simulink model "Kundur_BESS_STA_Nov14_2021a_v2_2021a"  (R2023a)
settings: Solver=VariableStepAuto  StartTime=0.0  StopTime=3  FixedStep=Ts  MaxStep=1e-5  MinStep=1e-20  RelTol=1e-3  EnableMultiTasking=on
PreLoadFcn:
  | Ts=50e-6;
PostLoadFcn:
  | Ts=50e-6;
InitFcn:
  | Ts=50e-6;
values from neighbouring files (symbols this model uses):
  current_K_den = [1 -1.95396088137 0.953960881373]    [param_cntrl_v2.mat]
  current_K_num = [292.549944556 -582.765243791 290.215658722]    [param_cntrl_v2.mat]
  flt_den = [1 -1.99914493247 0.999500180349]    [param_cntrl_v2.mat]
  flt_num = [0.000249925443627 3.12366678454e-08 -0.000249894206959]    [param_cntrl_v2.mat]
  flt_rocof_den = [1 -3.94812243331 5.84544117496 -3.84650440967 0.949185710471]    [param_cntrl_v2.mat]
  flt_rocof_num = [2.65341753303e-09 1.06136701321e-08 1.59205051982e-08 1.06136701321e-08 2.65341753303e-09]    [param_cntrl_v2.mat]
  pll_K_den = [1 -1.95396088137 0.953960881373]    [param_cntrl_v2.mat]
  pll_K_num = [1047.77474974 -2078.89023245 1031.12061217]    [param_cntrl_v2.mat]
  sampling_k = 5e-05    [param_cntrl_v2.mat]
undefined symbols (not defined in the file or in its folder): Ad2, Ad4, Bd2, Bd4, Cd2, Cd4, D1, Delta, flt_rocof_a_den, flt_rocof_a_num, flt_rocof_b_den, flt_rocof_b_num, Gd2, Gd4, Kd2, Kd4, L, R
libraries: spsThreePhaseVIMeasurementLib x15, spsLoadFlowBusLib x12, spsSeriesRLCBranchLib x11, spsThreePhaseSeriesRLCLoadLib x11, spsThreePhaseTransformerTwoWindingsLib x8, spsThreePhaseSeriesRLCBranchLib x8, spsabctoAlphaBetaZeroLib x8, spsGenericPowerSystemStabilizerLib x8, spsPowerPositiveSequenceLib x7, spsThreePhaseParallelRLCLoadLib x6, spsPLL3phLib x6, spsGroundLib x6
(part 4 of 4)

== system Kundur_BESS_STA_Nov14_2021a_v2_2021a/Area 2/sig1 ==
  In1 : Inport
  Bus Selector1 : BusSelector  OutputSignals="dq0 components.Stator voltage  vq (pu),dq0 components.Stator voltage  vd (pu),Mechanical.Rotor angle deviation  d_theta (rad),Mechanical.Rotor speed  wm  (pu),Mechanical.Electrical power  Pe (pu),Mechanical.Rotor speed deviation  dw (pu),Mechanical.Rotor mechanical angle  theta (deg)"
  Mux : Mux  Inputs=6
  Mux1 : Mux  Inputs=2
  Out1 : Outport  VectorParamsAs1DForOutWhenUnconnected=off
  wires:
  Mux1/1 -> Mux/1
  Bus Selector1/1 -> Mux1/1  "<Stator voltage  vq (pu)>"
  Bus Selector1/2 -> Mux1/2  "<Stator voltage  vd (pu)>"
  Bus Selector1/3 -> Mux/2  "<Rotor angle deviation  d_theta (rad)>"
  Bus Selector1/4 -> Mux/3  "<Rotor speed  wm  (pu)>"
  Bus Selector1/5 -> Mux/4  "<Electrical power  Pe (pu)>"
  Bus Selector1/6 -> Mux/5  "<Rotor speed deviation  dw (pu)>"
  Bus Selector1/7 -> Mux/6  "<Rotor mechanical angle  theta (deg)>"
  In1/1 -> Bus Selector1/1
  Mux/1 -> Out1/1

== system Kundur_BESS_STA_Nov14_2021a_v2_2021a/Area 2/sig2 ==
  In1 : Inport
  Bus Selector1 : BusSelector  OutputSignals="dq0 components.Stator voltage  vq (pu),dq0 components.Stator voltage  vd (pu),Mechanical.Rotor angle deviation  d_theta (rad),Mechanical.Rotor speed  wm  (pu),Mechanical.Electrical power  Pe (pu),Mechanical.Rotor speed deviation  dw (pu),Mechanical.Rotor mechanical angle  theta (deg)"
  Mux : Mux  Inputs=6
  Mux1 : Mux  Inputs=2
  Out1 : Outport  VectorParamsAs1DForOutWhenUnconnected=off
  wires:
  Mux1/1 -> Mux/1
  Bus Selector1/1 -> Mux1/1  "<Stator voltage  vq (pu)>"
  Bus Selector1/2 -> Mux1/2  "<Stator voltage  vd (pu)>"
  Bus Selector1/3 -> Mux/2  "<Rotor angle deviation  d_theta (rad)>"
  Bus Selector1/4 -> Mux/3  "<Rotor speed  wm  (pu)>"
  Bus Selector1/5 -> Mux/4  "<Electrical power  Pe (pu)>"
  Bus Selector1/6 -> Mux/5  "<Rotor speed deviation  dw (pu)>"
  Bus Selector1/7 -> Mux/6  "<Rotor mechanical angle  theta (deg)>"
  In1/1 -> Bus Selector1/1
  Mux/1 -> Out1/1

== system Kundur_BESS_STA_Nov14_2021a_v2_2021a/Area 1/BESS/Subsystem ==
  note: Alpha-Beta-Zero
      | to abc
  dq0 : Inport  PortDimensions=3
  wt1 : Inport  Port=2  PortDimensions=1
  Alpha-Beta-Zero to abc : spsAlphaBetaZerotoabcLib/Alpha-Beta-Zero to abc
  DQ to Alpha beta : Subsystem
  abc : Outport  VectorParamsAs1DForOutWhenUnconnected=off
  wires:
  Alpha-Beta-Zero to abc/1 -> abc/1
  dq0/1 -> DQ to Alpha beta/1(dq0)
  DQ to Alpha beta/1(al_be_0) -> Alpha-Beta-Zero to abc/1
  wt1/1 -> DQ to Alpha beta/2(wt1)

== system Kundur_BESS_STA_Nov14_2021a_v2_2021a/Area 1/BESS/Subsystem1 ==
  wt : Inport  PortDimensions=1
  abc : Inport  Port=2  PortDimensions=3
  Demux : Demux  Outputs=3
  Mux : Mux  Inputs=2
  Subsystem1 : Subsystem
  Terminator : Terminator
  abc to Alpha-Beta-Zero : spsabctoAlphaBetaZeroLib/abc to Alpha-Beta-Zero
  dq : Outport  VectorParamsAs1DForOutWhenUnconnected=off
  wires:
  Subsystem1/1(dq) -> dq/1
  abc/1 -> abc to Alpha-Beta-Zero/1
  wt/1 -> Subsystem1/2(wt1)
  Demux/1 -> Mux/1
  Demux/2 -> Mux/2
  Mux/1 -> Subsystem1/1(al_be)
  abc to Alpha-Beta-Zero/1 -> Demux/1
  Demux/3 -> Terminator/1

== system Kundur_BESS_STA_Nov14_2021a_v2_2021a/Area 1/BESS/Subsystem2 ==
  wt : Inport  PortDimensions=1
  abc : Inport  Port=2  PortDimensions=3
  Demux : Demux  Outputs=3
  Mux : Mux  Inputs=2
  Subsystem1 : Subsystem
  Terminator : Terminator
  abc to Alpha-Beta-Zero : spsabctoAlphaBetaZeroLib/abc to Alpha-Beta-Zero
  dq : Outport  VectorParamsAs1DForOutWhenUnconnected=off
  wires:
  Subsystem1/1(dq) -> dq/1
  abc/1 -> abc to Alpha-Beta-Zero/1
  wt/1 -> Subsystem1/2(wt1)
  Demux/1 -> Mux/1
  Demux/2 -> Mux/2
  Demux/3 -> Terminator/1
  Mux/1 -> Subsystem1/1(al_be)
  abc to Alpha-Beta-Zero/1 -> Demux/1

== system Kundur_BESS_STA_Nov14_2021a_v2_2021a/Area 1/BESS/Subsystem3 ==
  e(S) : Inport
  Add : Sum
  Integrator : Integrator
  Ki : Gain  Gain=Ki
  Kp : Gain  Gain=Kp
  u(S) : Outport  VectorParamsAs1DForOutWhenUnconnected=off
  wires:
  Kp/1 -> Add/1
  e(S)/1 -> Ki/1, Kp/1
  Ki/1 -> Integrator/1
  Add/1 -> u(S)/1  "u(S)"
  Integrator/1 -> Add/2

== system Kundur_BESS_STA_Nov14_2021a_v2_2021a/Area 1/BESS/Subsystem4 ==
  e(S) : Inport
  Add : Sum
  Integrator : Integrator
  Ki : Gain  Gain=Ki
  Kp : Gain  Gain=Kp
  u(S) : Outport  VectorParamsAs1DForOutWhenUnconnected=off
  wires:
  Kp/1 -> Add/1
  e(S)/1 -> Ki/1, Kp/1
  Ki/1 -> Integrator/1
  Add/1 -> u(S)/1  "u(S)"
  Integrator/1 -> Add/2

== system Kundur_BESS_STA_Nov14_2021a_v2_2021a/Area 1/BESS2 /Subsystem ==
  note: Alpha-Beta-Zero
      | to abc
  dq0 : Inport  PortDimensions=3
  wt1 : Inport  Port=2  PortDimensions=1
  Alpha-Beta-Zero to abc : spsAlphaBetaZerotoabcLib/Alpha-Beta-Zero to abc
  DQ to Alpha beta : Subsystem
  abc : Outport  VectorParamsAs1DForOutWhenUnconnected=off
  wires:
  Alpha-Beta-Zero to abc/1 -> abc/1
  dq0/1 -> DQ to Alpha beta/1(dq0)
  DQ to Alpha beta/1(al_be_0) -> Alpha-Beta-Zero to abc/1
  wt1/1 -> DQ to Alpha beta/2(wt1)

== system Kundur_BESS_STA_Nov14_2021a_v2_2021a/Area 1/BESS2 /Subsystem1 ==
  wt : Inport  PortDimensions=1
  abc : Inport  Port=2  PortDimensions=3
  Demux : Demux  Outputs=3
  Mux : Mux  Inputs=2
  Subsystem1 : Subsystem
  Terminator : Terminator
  abc to Alpha-Beta-Zero : spsabctoAlphaBetaZeroLib/abc to Alpha-Beta-Zero
  dq : Outport  VectorParamsAs1DForOutWhenUnconnected=off
  wires:
  Subsystem1/1(dq) -> dq/1
  abc/1 -> abc to Alpha-Beta-Zero/1
  wt/1 -> Subsystem1/2(wt1)
  Demux/1 -> Mux/1
  Demux/2 -> Mux/2
  Mux/1 -> Subsystem1/1(al_be)
  abc to Alpha-Beta-Zero/1 -> Demux/1
  Demux/3 -> Terminator/1

== system Kundur_BESS_STA_Nov14_2021a_v2_2021a/Area 1/BESS2 /Subsystem2 ==
  wt : Inport  PortDimensions=1
  abc : Inport  Port=2  PortDimensions=3
  Demux : Demux  Outputs=3
  Mux : Mux  Inputs=2
  Subsystem1 : Subsystem
  Terminator : Terminator
  abc to Alpha-Beta-Zero : spsabctoAlphaBetaZeroLib/abc to Alpha-Beta-Zero
  dq : Outport  VectorParamsAs1DForOutWhenUnconnected=off
  wires:
  Subsystem1/1(dq) -> dq/1
  abc/1 -> abc to Alpha-Beta-Zero/1
  wt/1 -> Subsystem1/2(wt1)
  Demux/1 -> Mux/1
  Demux/2 -> Mux/2
  Demux/3 -> Terminator/1
  Mux/1 -> Subsystem1/1(al_be)
  abc to Alpha-Beta-Zero/1 -> Demux/1

== system Kundur_BESS_STA_Nov14_2021a_v2_2021a/Area 1/BESS2 /Subsystem3 ==
  e(S) : Inport
  Add : Sum
  Integrator : Integrator
  Ki : Gain  Gain=Ki
  Kp : Gain  Gain=Kp
  u(S) : Outport  VectorParamsAs1DForOutWhenUnconnected=off
  wires:
  Kp/1 -> Add/1
  e(S)/1 -> Ki/1, Kp/1
  Ki/1 -> Integrator/1
  Add/1 -> u(S)/1  "u(S)"
  Integrator/1 -> Add/2

== system Kundur_BESS_STA_Nov14_2021a_v2_2021a/Area 1/BESS2 /Subsystem4 ==
  e(S) : Inport
  Add : Sum
  Integrator : Integrator
  Ki : Gain  Gain=Ki
  Kp : Gain  Gain=Kp
  u(S) : Outport  VectorParamsAs1DForOutWhenUnconnected=off
  wires:
  Kp/1 -> Add/1
  e(S)/1 -> Ki/1, Kp/1
  Ki/1 -> Integrator/1
  Add/1 -> u(S)/1  "u(S)"
  Integrator/1 -> Add/2

== system Kundur_BESS_STA_Nov14_2021a_v2_2021a/Area 2/BESS/Aver. Inverter ==
  U_abc : Inport
  Controlled Voltage Source : spsControlledVoltageSourceLib/Controlled Voltage Source  Initialize=on  Source_Type=AC  Amplitude=0  Phase=0  Frequency=0  Measurements=None
  Controlled Voltage Source1 : spsControlledVoltageSourceLib/Controlled Voltage Source  Initialize=on  Source_Type=AC  Amplitude=0  Phase=0  Frequency=0  Measurements=None
  Controlled Voltage Source2 : spsControlledVoltageSourceLib/Controlled Voltage Source  Initialize=on  Source_Type=AC  Amplitude=0  Phase=0  Frequency=0  Measurements=None
  Demux : Demux  Outputs=3
  Ground : spsGroundLib/Ground  LConnTagsString=a
  A : PMIOPort  Side=Right
  B : PMIOPort  Port=2  Side=Right
  C : PMIOPort  Port=3  Side=Right
  wires:
  Demux/1 -> Controlled Voltage Source/1
  Demux/2 -> Controlled Voltage Source1/1
  Demux/3 -> Controlled Voltage Source2/1
  U_abc/1 -> Demux/1
  connections:
  Controlled Voltage Source/LConn1 -- Controlled Voltage Source1/LConn1 -- Controlled Voltage Source2/LConn1 -- Ground/LConn1
  Controlled Voltage Source2/RConn1 -- C/RConn1
  Controlled Voltage Source1/RConn1 -- B/RConn1
  Controlled Voltage Source/RConn1 -- A/RConn1

== system Kundur_BESS_STA_Nov14_2021a_v2_2021a/Area 2/BESS/I_ref ==
  note: Ud^2+Uq^2
  note: [Uq;Ud]
  note: [Ud;-Uq]
  PQ : Inport
  U_dq0 : Inport  Port=2
  Constant : Constant  Value=0
  Divide : Product  Inputs=*/
  Divide1 : Product  Inputs=*/
  Dot Product : DotProduct  OutDataTypeStr=Inherit: Inherit via internal rule
  Dot Product1 : DotProduct  OutDataTypeStr=Inherit: Inherit via internal rule
  Dot Product2 : DotProduct  OutDataTypeStr=Inherit: Inherit via internal rule
  Gain : Gain  Gain=[1,0;0,-1]  Multiplication=Matrix(K*u)
  Gain1 : Gain  Gain=[0,1;1,0]  Multiplication=Matrix(K*u)
  Gain2 : Gain  Gain=2/3
  Gain3 : Gain  Gain=2/3
  Mux : Mux  Inputs=3
  Saturation : Saturate  UpperLimit=1e10  LowerLimit=1e-4
  Selector : Selector  InputPortWidth=3  IndexOptions=Index vector (dialog)  Indices=[1 2]  OutputSizes=1
  I_dq0_ref : Outport
  wires:
  U_dq0/1 -> Selector/1
  Selector/1 -> Dot Product2/1, Dot Product2/2, Gain1/1, Gain/1
  Gain/1 -> Dot Product/2
  Gain1/1 -> Dot Product1/2
  PQ/1 -> Dot Product/1, Dot Product1/1
  Dot Product/1 -> Divide/1
  Dot Product1/1 -> Divide1/1
  Divide/1 -> Gain2/1
  Divide1/1 -> Gain3/1
  Mux/1 -> I_dq0_ref/1
  Constant/1 -> Mux/3
  Dot Product2/1 -> Saturation/1
  Saturation/1 -> Divide1/2, Divide/2
  Gain2/1 -> Mux/1
  Gain3/1 -> Mux/2

== system Kundur_BESS_STA_Nov14_2021a_v2_2021a/Area 2/BESS/SRF-PLL1 ==
  Uabc : Inport
  Alpha-Beta-Zero to dq0 : spsAlphaBetaZerotodq0Lib/Alpha-Beta-Zero to dq0  Alignment=Aligned with phase A axis
  Constant1 : Constant  Value=60*2*pi
  DSOGI : Subsystem  Commented=on
      settings: PortSchema="{\"entries\":[{\"content\":{\"sides\":[{\"content\":{\"connectorIds\":[\"In1\"]},\"type\":\"ConnectorPlacement.EquallySpacedRectSide\",\"uuid\":\"0e58ca25-f6ec-443d-b264-f69bb116b758\"},{\"content\":{\"connectorIds\":[\"Out1\"],\"side\":\"RIGHT\"},\"type\":\"ConnectorPlacement.EquallySpacedRectSide\",\"uuid\":\"f4052289-4772-41c6-aa5a-e32d1aa36c69\"},{\"content\":{\"side\":\"TOP\"},\"type\":\"ConnectorPlacement.EquallySpacedRectSide\",\"uuid\":\"ea46d89b-d5cb-4111-9a8a-24f542a45993\"},{\"content\":{\"connectorIds\":[\"In2\"],\"side\":\"BOTTOM\"},\"type\":\"ConnectorPlacement.EquallySpacedRectSide\",\"uuid\":\"bc0e78b7-d9b3-48dd-a6ae-aa9871795585\"}]},\"type\":\"ConnectorPlacement.EquallySpacedConnector\",\"uuid\":\"463a5158-fade-4a5a-b60d-59d7cf065d44\"}],\"packageUris\":[\"http://schema.mathworks.com/mf0/Connector/R2020b\"],\"version\":\"1.0\"}"
  Discrete Transfer Fcn : DiscreteTransferFcn  Numerator=pll_K_num  Denominator=pll_K_den
  Filter : Subsystem  Commented=on
  Gain : Gain  Gain=sampling_k
  Normalization : dspmathops/Normalization  NormType=2-norm  Bias=1e-10  NormOver=Each column  Dimension=1  roundingMode=Floor  overflowMode=off  accumDataTypeStr=Inherit: Same as product output  accumLastDataTypeStr=Inherit: Same as product output  outputDataTypeStr=Inherit: Same as product output  outputMin=[]  outputMax=[]  outputLastDataTypeStr=Inherit: Same as product output
  Quadrature : Subsystem
  Scope : Scope
  Selector : Selector  InputPortWidth=3  IndexOptions=Index vector (dialog)  Indices=2  OutputSizes=1
  Sum : Sum  Inputs=++|
  Sum2 : Sum  Inputs=++|
  Unit Delay : UnitDelay  SampleTime=sampling_k  HasFrameUpgradeWarning=on
  Wrap : Subsystem
  filt : Subsystem
  w : Outport
  ph : Outport  Port=2
  wires:
  Sum/1 -> Unit Delay/1
  Gain/1 -> Sum/2
  Unit Delay/1 -> Wrap/1(phi)
  Selector/1 -> Scope/1, Discrete Transfer Fcn/1
  Discrete Transfer Fcn/1 -> Sum2/2
  Sum2/1 -> filt/1(u), Gain/1
  Constant1/1 -> Sum2/1
  Alpha-Beta-Zero to dq0/1 -> Selector/1
  Normalization/1 -> Alpha-Beta-Zero to dq0/1
  Quadrature/1(Ualphbet0) -> Normalization/1
  Uabc/1 -> Quadrature/1(Uabc)
  filt/1(uf) -> Quadrature/2(w), w/1
  Wrap/1(w_phi) -> ph/1, Alpha-Beta-Zero to dq0/2, Sum/1

== system Kundur_BESS_STA_Nov14_2021a_v2_2021a/Area 2/BESS/Support Control ==
  note: 1) Add Subsystem or Model blocks as valid variant choices.
      | 2) You cannot connect blocks at this level. At simulation, connectivity is automatically
      | determined, based on the active variant and port name matching.
  Vabc : Inport
  Gains : Inport  Port=2
  Droop (Proportional) : Subsystem  VariantControl=false
  VI with Diff : Subsystem  VariantControl=false
  VI with STA : Subsystem  VariantControl=true
  P_ref : Outport

== system Kundur_BESS_STA_Nov14_2021a_v2_2021a/Area 2/BESS/abc-to-dq0 ==
  Uabc : Inport
  Iabc : Inport  Port=2
  wt : Inport  Port=3
  abc to dq2 : spsabctodq0Lib/abc to dq0  Alignment=90 degrees behind phase A axis
  abc to dq3 : spsabctodq0Lib/abc to dq0  Alignment=90 degrees behind phase A axis
  Udq0 : Outport
  Idq0 : Outport  Port=2
  wires:
  wt/1 -> abc to dq3/2, abc to dq2/2
  Iabc/1 -> abc to dq3/1
  Uabc/1 -> abc to dq2/1
  abc to dq2/1 -> Udq0/1
  abc to dq3/1 -> Idq0/1

== system Kundur_BESS_STA_Nov14_2021a_v2_2021a/Area 1/BESS/Subsystem/DQ to Alpha beta ==
  dq0 : Inport  PortDimensions=3
  wt1 : Inport  Port=2  PortDimensions=1
  Demux4 : Demux  Outputs=[2 1]
  Fcn : Fcn  Expr=u[1]*sin(u[3]) + u[2]*cos(u[3])
  Fcn1 : Fcn  Expr=-u[1]*cos(u[3]) + u[2]*sin(u[3])
  Mux1 : Mux  Inputs=[2 1]
  Mux4 : Mux  Inputs=2
  Mux5 : Mux  Inputs=[2 1]
  Mux6 : Mux  Inputs=[2 1]
  al_be_0 : Outport  VectorParamsAs1DForOutWhenUnconnected=off
  wires:
  Mux4/1 -> Mux1/1
  Mux6/1 -> Fcn1/1
  Fcn1/1 -> Mux4/2
  Demux4/1 -> Mux6/1, Mux5/1
  Mux5/1 -> Fcn/1
  Demux4/2 -> Mux1/2
  Fcn/1 -> Mux4/1
  wt1/1 -> Mux5/2, Mux6/2
  dq0/1 -> Demux4/1
  Mux1/1 -> al_be_0/1

== system Kundur_BESS_STA_Nov14_2021a_v2_2021a/Area 1/BESS/Subsystem1/Subsystem1 ==
  note: q = al*cos(wt) + be*sin(wt)
  note: d = al*sin(wt) - be*cos(wt)
  al_be : Inport  PortDimensions=2
  wt1 : Inport  Port=2  PortDimensions=1
  Fcn : Fcn  Expr=u[1]*sin(u[3]) - u[2]*cos(u[3])
  Fcn1 : Fcn  Expr=u[1]*cos(u[3]) + u[2]*sin(u[3])
  Mux4 : Mux  Inputs=2
  Mux5 : Mux  Inputs=[2 1]
  Mux6 : Mux  Inputs=[2 1]
  dq : Outport  VectorParamsAs1DForOutWhenUnconnected=off
  wires:
  Mux5/1 -> Fcn/1
  Fcn1/1 -> Mux4/2
  al_be/1 -> Mux6/1, Mux5/1
  wt1/1 -> Mux5/2, Mux6/2
  Mux6/1 -> Fcn1/1
  Fcn/1 -> Mux4/1
  Mux4/1 -> dq/1

== system Kundur_BESS_STA_Nov14_2021a_v2_2021a/Area 1/BESS/Subsystem2/Subsystem1 ==
  note: q = al*cos(wt) + be*sin(wt)
  note: d = al*sin(wt) - be*cos(wt)
  al_be : Inport  PortDimensions=2
  wt1 : Inport  Port=2  PortDimensions=1
  Fcn : Fcn  Expr=u[1]*sin(u[3]) - u[2]*cos(u[3])
  Fcn1 : Fcn  Expr=u[1]*cos(u[3]) + u[2]*sin(u[3])
  Mux4 : Mux  Inputs=2
  Mux5 : Mux  Inputs=[2 1]
  Mux6 : Mux  Inputs=[2 1]
  dq : Outport  VectorParamsAs1DForOutWhenUnconnected=off
  wires:
  Mux5/1 -> Fcn/1
  Fcn1/1 -> Mux4/2
  al_be/1 -> Mux6/1, Mux5/1
  wt1/1 -> Mux5/2, Mux6/2
  Mux6/1 -> Fcn1/1
  Fcn/1 -> Mux4/1
  Mux4/1 -> dq/1

== system Kundur_BESS_STA_Nov14_2021a_v2_2021a/Area 1/BESS2 /Subsystem/DQ to Alpha beta ==
  dq0 : Inport  PortDimensions=3
  wt1 : Inport  Port=2  PortDimensions=1
  Demux4 : Demux  Outputs=[2 1]
  Fcn : Fcn  Expr=u[1]*sin(u[3]) + u[2]*cos(u[3])
  Fcn1 : Fcn  Expr=-u[1]*cos(u[3]) + u[2]*sin(u[3])
  Mux1 : Mux  Inputs=[2 1]
  Mux4 : Mux  Inputs=2
  Mux5 : Mux  Inputs=[2 1]
  Mux6 : Mux  Inputs=[2 1]
  al_be_0 : Outport  VectorParamsAs1DForOutWhenUnconnected=off
  wires:
  Mux4/1 -> Mux1/1
  Mux6/1 -> Fcn1/1
  Fcn1/1 -> Mux4/2
  Demux4/1 -> Mux6/1, Mux5/1
  Mux5/1 -> Fcn/1
  Demux4/2 -> Mux1/2
  Fcn/1 -> Mux4/1
  wt1/1 -> Mux5/2, Mux6/2
  dq0/1 -> Demux4/1
  Mux1/1 -> al_be_0/1

== system Kundur_BESS_STA_Nov14_2021a_v2_2021a/Area 1/BESS2 /Subsystem1/Subsystem1 ==
  note: q = al*cos(wt) + be*sin(wt)
  note: d = al*sin(wt) - be*cos(wt)
  al_be : Inport  PortDimensions=2
  wt1 : Inport  Port=2  PortDimensions=1
  Fcn : Fcn  Expr=u[1]*sin(u[3]) - u[2]*cos(u[3])
  Fcn1 : Fcn  Expr=u[1]*cos(u[3]) + u[2]*sin(u[3])
  Mux4 : Mux  Inputs=2
  Mux5 : Mux  Inputs=[2 1]
  Mux6 : Mux  Inputs=[2 1]
  dq : Outport  VectorParamsAs1DForOutWhenUnconnected=off
  wires:
  Mux5/1 -> Fcn/1
  Fcn1/1 -> Mux4/2
  al_be/1 -> Mux6/1, Mux5/1
  wt1/1 -> Mux5/2, Mux6/2
  Mux6/1 -> Fcn1/1
  Fcn/1 -> Mux4/1
  Mux4/1 -> dq/1

== system Kundur_BESS_STA_Nov14_2021a_v2_2021a/Area 1/BESS2 /Subsystem2/Subsystem1 ==
  note: q = al*cos(wt) + be*sin(wt)
  note: d = al*sin(wt) - be*cos(wt)
  al_be : Inport  PortDimensions=2
  wt1 : Inport  Port=2  PortDimensions=1
  Fcn : Fcn  Expr=u[1]*sin(u[3]) - u[2]*cos(u[3])
  Fcn1 : Fcn  Expr=u[1]*cos(u[3]) + u[2]*sin(u[3])
  Mux4 : Mux  Inputs=2
  Mux5 : Mux  Inputs=[2 1]
  Mux6 : Mux  Inputs=[2 1]
  dq : Outport  VectorParamsAs1DForOutWhenUnconnected=off
  wires:
  Mux5/1 -> Fcn/1
  Fcn1/1 -> Mux4/2
  al_be/1 -> Mux6/1, Mux5/1
  wt1/1 -> Mux5/2, Mux6/2
  Mux6/1 -> Fcn1/1
  Fcn/1 -> Mux4/1
  Mux4/1 -> dq/1

== system Kundur_BESS_STA_Nov14_2021a_v2_2021a/Area 2/BESS/SRF-PLL1/DSOGI ==
  Uabc : Inport
  w(t) : Inport  Port=2
  Constant : Constant  Value=0
  Gain : Gain  Gain=1/1000
  Gain1 : Gain  Gain=0.01
  Gain2 : Gain  Gain=0.01
  Integrator{,1..3} (4 alike) : Integrator
  Mux : Mux  Inputs=3
  Product{,1..3} (4 alike) : Product
  Selector1 : Selector  InputPortWidth=3  IndexOptions=Index vector (dialog)  Indices=1  OutputSizes=1
  Selector2 : Selector  InputPortWidth=3  IndexOptions=Index vector (dialog)  Indices=2  OutputSizes=1
  Sum1 : Sum  Inputs=-+|
  Sum2 : Sum  Inputs=|+-
  Sum3 : Sum  Inputs=-+|
  Sum4 : Sum  Inputs=|+-
  Sum5 : Sum  Inputs=|+-
  Sum6 : Sum  Inputs=|++
  Zero-Order Hold2 : ZeroOrderHold  SampleTime=sampling_k
  abc to Alpha-Beta-Zero : spsabctoAlphaBetaZeroLib/abc to Alpha-Beta-Zero
  Ualphbet0 : Outport
  wires:
  Sum4/1 -> Product/2
  Selector1/1 -> Sum1/2
  Gain/1 -> Selector2/1, Selector1/1
  Gain1/1 -> Sum4/1
  Sum1/1 -> Gain1/1
  Uabc/1 -> abc to Alpha-Beta-Zero/1
  Product/1 -> Integrator/1
  Product1/1 -> Integrator1/1
  Integrator1/1 -> [qv_alpha], Sum4/2
  Integrator/1 -> Product1/2, [v_alpha], Sum1/1, Sum2/1
  w(t)/1 -> Product2/1, Product3/1, Product1/1, Product/1
  Selector2/1 -> Sum3/2
  Sum3/1 -> Gain2/1
  Gain2/1 -> Sum5/1
  Sum5/1 -> Product2/2
  Product2/1 -> Integrator2/1
  Integrator2/1 -> [v_beta], Product3/2, Sum3/1, Sum6/1
  Product3/1 -> Integrator3/1
  Integrator3/1 -> [qv_beta], Sum5/2
  Sum2/1 -> Mux/1
  Sum6/1 -> Mux/2
  Constant/1 -> Mux/3
  Mux/1 -> Zero-Order Hold2/1
  Zero-Order Hold2/1 -> Ualphbet0/1
  abc to Alpha-Beta-Zero/1 -> Gain/1
  [qv_beta] -> Sum2/2
  [qv_alpha] -> Sum6/2

== system Kundur_BESS_STA_Nov14_2021a_v2_2021a/Area 2/BESS/SRF-PLL1/Filter ==
  Uabc : Inport
  Demux : Demux  Outputs=3
  Discrete Transfer Fcn : DiscreteTransferFcn  Numerator=flt_num  Denominator=flt_den
  Discrete Transfer Fcn1 : DiscreteTransferFcn  Numerator=flt_num  Denominator=flt_den
  Discrete Transfer Fcn2 : DiscreteTransferFcn  Numerator=flt_num  Denominator=flt_den
  Mux : Mux  Inputs=3
  Zero-Order Hold1 : ZeroOrderHold  SampleTime=sampling_k
  Zero-Order Hold2 : ZeroOrderHold  SampleTime=sampling_k
  Zero-Order Hold3 : ZeroOrderHold  SampleTime=sampling_k
  Uabc_f : Outport
  wires:
  Uabc/1 -> Demux/1
  Mux/1 -> Uabc_f/1
  Demux/1 -> Zero-Order Hold2/1
  Demux/2 -> Zero-Order Hold1/1
  Demux/3 -> Zero-Order Hold3/1
  Zero-Order Hold2/1 -> Discrete Transfer Fcn/1
  Zero-Order Hold1/1 -> Discrete Transfer Fcn1/1
  Zero-Order Hold3/1 -> Discrete Transfer Fcn2/1
  Discrete Transfer Fcn/1 -> Mux/1
  Discrete Transfer Fcn1/1 -> Mux/2
  Discrete Transfer Fcn2/1 -> Mux/3

== system Kundur_BESS_STA_Nov14_2021a_v2_2021a/Area 2/BESS/SRF-PLL1/Quadrature ==
  Uabc : Inport
  w : Inport  Port=2
  Constant : Constant  Value=0
  Divide : Product  Inputs=*/
  Gain : Gain  Gain=1/1000
  Mux : Mux  Inputs=3
  Saturation : Saturate  UpperLimit=62*2*pi  LowerLimit=59*2*pi
  Scope1 : Scope  NumInputPorts=2
  Selector : Selector  InputPortWidth=3  IndexOptions=Index vector (dialog)  Indices=1  OutputSizes=1
  State-Space : StateSpace  A=[-42e3,1,0;-586e6,0,1;-2712e9,0,0]  B=[42e3;586e6;2712e9]  C=[0,1,0]  D=[0]  InitialCondition=0
  Transfer Fcn1 : TransferFcn  Denominator=[1/(1200*2*pi)^2,2*0.1/(1200*2*pi),1]
  Zero-Order Hold2 : ZeroOrderHold  SampleTime=sampling_k
  abc to Alpha-Beta-Zero : spsabctoAlphaBetaZeroLib/abc to Alpha-Beta-Zero
  Ualphbet0 : Outport
  wires:
  Uabc/1 -> Gain/1
  Gain/1 -> abc to Alpha-Beta-Zero/1
  Zero-Order Hold2/1 -> Ualphbet0/1
  abc to Alpha-Beta-Zero/1 -> Selector/1
  Constant/1 -> Mux/3
  Mux/1 -> Zero-Order Hold2/1
  Transfer Fcn1/1 -> Scope1/2, Mux/2, State-Space/1
  State-Space/1 -> Divide/1
  w/1 -> Saturation/1
  Saturation/1 -> Divide/2
  Divide/1 -> Scope1/1, Mux/1
  Selector/1 -> Transfer Fcn1/1

== system Kundur_BESS_STA_Nov14_2021a_v2_2021a/Area 2/BESS/SRF-PLL1/Wrap ==
  phi : Inport
  Constant : Constant  Value=pi
  Constant1 : Constant  Value=2*pi
  Divide : Product  Inputs=*/
  Floor : Rounding
  Product : Product
  Sum : Sum  Inputs=|+-
  Sum1 : Sum  Inputs=|+-
  Sum2 : Sum  Inputs=|+-
  w_phi : Outport
  wires:
  phi/1 -> Sum/1
  Constant/1 -> Sum2/2, Sum/2
  Sum/1 -> Divide/1, Sum1/1
  Constant1/1 -> Product/2, Divide/2
  Divide/1 -> Floor/1
  Floor/1 -> Product/1
  Product/1 -> Sum1/2
  Sum1/1 -> Sum2/1
  Sum2/1 -> w_phi/1

== system Kundur_BESS_STA_Nov14_2021a_v2_2021a/Area 2/BESS/SRF-PLL1/filt ==
  u : Inport
  Discrete Transfer Fcn1 : DiscreteTransferFcn  Numerator=flt_rocof_num  Denominator=flt_rocof_den
  Discrete Transfer Fcn2 : DiscreteTransferFcn  Numerator=flt_rocof_num  Denominator=flt_rocof_den
  uf : Outport
  wires:
  u/1 -> Discrete Transfer Fcn1/1
  Discrete Transfer Fcn1/1 -> Discrete Transfer Fcn2/1
  Discrete Transfer Fcn2/1 -> uf/1

== system Kundur_BESS_STA_Nov14_2021a_v2_2021a/Area 2/BESS/Support Control/Droop (Proportional) ==
  Vabc : Inport
  Gains : Inport  Port=2
  Gain : Gain  Gain=-1
  PLL (3ph) : spsPLL3phLib/PLL (3ph)  Fmin=45  Par_Init=[0, 50]  ParK=[180, 3200, 0]  TcD=1e-4  MaxRateChangeFreq=12  FilterCutOffFreq=25  Ts=0  AGC=on
  Product : Product
  Selector : Selector  InputPortWidth=3  IndexOptions=Index vector (dialog)  Indices=1  OutputSizes=1
  Selector1 : Selector  InputPortWidth=3  IndexOptions=Index vector (dialog)  Indices=3  OutputSizes=1
  Sum : Sum  Inputs=-+|
  Terminator : Terminator
  P_ref : Outport
  wires:
  Vabc/1 -> PLL (3ph)/1
  Gains/1 -> Selector1/1, Selector/1
  PLL (3ph)/1 -> Sum/2  "freq"
  Selector1/1 -> Sum/1  "freq 0"
  PLL (3ph)/2 -> Terminator/1
  Sum/1 -> Product/2
  Selector/1 -> Product/1  "K_P"
  Product/1 -> Gain/1
  Gain/1 -> P_ref/1

== system Kundur_BESS_STA_Nov14_2021a_v2_2021a/Area 2/BESS/Support Control/VI with Diff ==
  Vabc : Inport
  Gains : Inport  Port=2
  Diff : TransferFcn  Numerator=[1 0]  Denominator=[0.005 1]
  Filter : TransferFcn  Denominator=[0.3 1]
  Gain : Gain  Gain=-1
  PLL (3ph) : spsPLL3phLib/PLL (3ph)  Fmin=45  Par_Init=[0, 50]  ParK=[180, 3200, 0]  TcD=1e-4  MaxRateChangeFreq=12  FilterCutOffFreq=25  Ts=0  AGC=on
  Product : Product
  Product1 : Product
  Selector : Selector  InputPortWidth=3  IndexOptions=Index vector (dialog)  Indices=1  OutputSizes=1
  Selector1 : Selector  InputPortWidth=3  IndexOptions=Index vector (dialog)  Indices=3  OutputSizes=1
  Selector2 : Selector  InputPortWidth=3  IndexOptions=Index vector (dialog)  Indices=2  OutputSizes=1
  Sum : Sum  Inputs=-+|
  Sum1 : Sum  Inputs=|++
  Terminator : Terminator
  P_ref : Outport
  wires:
  Gain/1 -> P_ref/1
  Selector/1 -> Product/1  "K_P"
  Sum/1 -> Filter/1, Product/2
  PLL (3ph)/2 -> Terminator/1
  Selector1/1 -> Sum/1  "freq 0"
  PLL (3ph)/1 -> Sum/2  "freq"
  Gains/1 -> Selector2/1, Selector/1, Selector1/1
  Vabc/1 -> PLL (3ph)/1
  Selector2/1 -> Product1/1  "K_D"
  Product/1 -> Sum1/1
  Sum1/1 -> Gain/1
  Filter/1 -> Diff/1
  Diff/1 -> Product1/2
  Product1/1 -> Sum1/2

== system Kundur_BESS_STA_Nov14_2021a_v2_2021a/Area 2/BESS/Support Control/VI with STA ==
  Vabc : Inport
  Gains : Inport  Port=2
  Dead Zone : DeadZone  LowerValue=-8e-3  UpperValue=8e-3
  Dead Zone1 : DeadZone  LowerValue=-0.25  UpperValue=0.25
  Demux : Demux  Outputs=3
  Mux : Mux  Inputs=2
  Mux1 : Mux  Inputs=2
  Product : Product
  Product1 : Product
  STA-PLL : Subsystem
  Scope1 : Scope  NumInputPorts=2
  Scope2 : Scope
  Sum : Sum  Inputs=-+|
  Sum1 : Sum  Inputs=|--
  P_ref : Outport
  wires:
  Gains/1 -> Demux/1
  Vabc/1 -> STA-PLL/1(V_abc)
  STA-PLL/1(Freq) -> Scope2/1, Sum/2
  Demux/3 -> Sum/1
  Demux/1 -> Product/1
  STA-PLL/2(RoCoF) -> Mux1/1, Dead Zone1/1
  Demux/2 -> Product1/2
  Product/1 -> Sum1/1
  Product1/1 -> Sum1/2
  Sum/1 -> Mux/1, Dead Zone/1
  Dead Zone/1 -> Mux/2, Product/2
  Dead Zone1/1 -> Mux1/2, Product1/1
  Sum1/1 -> P_ref/1
  Mux/1 -> Scope1/1
  Mux1/1 -> Scope1/2

== system Kundur_BESS_STA_Nov14_2021a_v2_2021a/Area 2/BESS/Support Control/VI with STA/STA-PLL ==
  V_abc : Inport
  2pi1 : Gain  Gain=1/2/pi
  2pi4 : Gain  Gain=1/2/pi
  Alpha-Beta-Zero to dq0 : spsAlphaBetaZerotodq0Lib/Alpha-Beta-Zero to dq0  Alignment=Aligned with phase A axis
  DSOGI : Subsystem  Commented=on
      settings: PortSchema="{\"entries\":[{\"content\":{\"sides\":[{\"content\":{\"connectorIds\":[\"In1\"]},\"type\":\"ConnectorPlacement.EquallySpacedRectSide\",\"uuid\":\"0e58ca25-f6ec-443d-b264-f69bb116b758\"},{\"content\":{\"connectorIds\":[\"Out1\"],\"side\":\"RIGHT\"},\"type\":\"ConnectorPlacement.EquallySpacedRectSide\",\"uuid\":\"f4052289-4772-41c6-aa5a-e32d1aa36c69\"},{\"content\":{\"side\":\"TOP\"},\"type\":\"ConnectorPlacement.EquallySpacedRectSide\",\"uuid\":\"ea46d89b-d5cb-4111-9a8a-24f542a45993\"},{\"content\":{\"connectorIds\":[\"In2\"],\"side\":\"BOTTOM\"},\"type\":\"ConnectorPlacement.EquallySpacedRectSide\",\"uuid\":\"bc0e78b7-d9b3-48dd-a6ae-aa9871795585\"}]},\"type\":\"ConnectorPlacement.EquallySpacedConnector\",\"uuid\":\"463a5158-fade-4a5a-b60d-59d7cf065d44\"}],\"packageUris\":[\"http://schema.mathworks.com/mf0/Connector/R2020b\"],\"version\":\"1.0\"}"
  Gain : Gain  Gain=sampling_k
  Gain2 : Gain  Gain=sampling_k
  Normalization : dspmathops/Normalization  NormType=2-norm  Bias=1e-10  NormOver=Each column  Dimension=1  roundingMode=Floor  overflowMode=off  accumDataTypeStr=Inherit: Same as product output  accumLastDataTypeStr=Inherit: Same as product output  outputDataTypeStr=Inherit: Same as product output  outputMin=[]  outputMax=[]  outputLastDataTypeStr=Inherit: Same as product output
  Quadrature : Subsystem
  Scope : Scope  NumInputPorts=2
  Scope2 : Scope
  Scope3 : Scope
  Selector : Selector  InputPortWidth=3  IndexOptions=Index vector (dialog)  Indices=2  OutputSizes=1
  Sign : Signum
  Signed Sqrt : Sqrt  Operator=signedSqrt
  Sum : Sum  Inputs=++|
  Sum2 : Sum  Inputs=|++
  Sum3 : Sum  Inputs=++|
  Unit Delay : UnitDelay  SampleTime=sampling_k  HasFrameUpgradeWarning=on
  Unit Delay2 : UnitDelay  InitialCondition=60*2*pi  SampleTime=sampling_k  HasFrameUpgradeWarning=on
  Wrap : Subsystem
  filt1 : Subsystem
  filt3 : Subsystem
  filt4 : Subsystem  Commented=on
  k1 : Gain  Gain=-35
  k2 : Gain  Gain=-30
  Freq : Outport
  RoCoF : Outport  Port=2
  wires:
  Normalization/1 -> Alpha-Beta-Zero to dq0/1, Scope3/1
  Unit Delay/1 -> Wrap/1(phi)
  Gain/1 -> Sum/2
  Wrap/1(w_phi) -> Alpha-Beta-Zero to dq0/2, Sum/1
  Sum/1 -> Unit Delay/1
  Unit Delay2/1 -> Scope/2, Sum2/2, Sum3/1
  Selector/1 -> Signed Sqrt/1, Sign/1, Scope2/1
  Sum3/1 -> Unit Delay2/1
  k1/1 -> Sum2/1
  k2/1 -> filt1/1(u), Gain2/1
  Signed Sqrt/1 -> k1/1
  Gain2/1 -> Sum3/2
  Sign/1 -> k2/1
  Sum2/1 -> filt3/1(u), Scope/1, Gain/1
  Alpha-Beta-Zero to dq0/1 -> Selector/1
  2pi1/1 -> RoCoF/1
  V_abc/1 -> Quadrature/1(Uabc)
  Quadrature/1(Ualphbet0) -> Normalization/1
  filt3/1(uf) -> 2pi4/1, Quadrature/2(w)
  filt1/1(uf) -> 2pi1/1
  2pi4/1 -> Freq/1

== system Kundur_BESS_STA_Nov14_2021a_v2_2021a/Area 2/BESS/Support Control/VI with STA/STA-PLL/DSOGI ==
  Uabc : Inport
  w(t) : Inport  Port=2
  Constant : Constant  Value=0
  Gain : Gain  Gain=1/1000
  Gain1 : Gain  Gain=0.01
  Gain2 : Gain  Gain=0.01
  Integrator{,1..3} (4 alike) : Integrator
  Mux : Mux  Inputs=3
  Product{,1..3} (4 alike) : Product
  Selector1 : Selector  InputPortWidth=3  IndexOptions=Index vector (dialog)  Indices=1  OutputSizes=1
  Selector2 : Selector  InputPortWidth=3  IndexOptions=Index vector (dialog)  Indices=2  OutputSizes=1
  Sum1 : Sum  Inputs=-+|
  Sum2 : Sum  Inputs=|+-
  Sum3 : Sum  Inputs=-+|
  Sum4 : Sum  Inputs=|+-
  Sum5 : Sum  Inputs=|+-
  Sum6 : Sum  Inputs=|++
  Zero-Order Hold2 : ZeroOrderHold  SampleTime=sampling_k
  abc to Alpha-Beta-Zero : spsabctoAlphaBetaZeroLib/abc to Alpha-Beta-Zero
  Ualphbet0 : Outport
  wires:
  Sum4/1 -> Product/2
  Selector1/1 -> Sum1/2
  Gain/1 -> Selector2/1, Selector1/1
  Gain1/1 -> Sum4/1
  Sum1/1 -> Gain1/1
  Uabc/1 -> abc to Alpha-Beta-Zero/1
  Product/1 -> Integrator/1
  Product1/1 -> Integrator1/1
  Integrator1/1 -> [qv_alpha], Sum4/2
  Integrator/1 -> Product1/2, [v_alpha], Sum1/1, Sum2/1
  w(t)/1 -> Product2/1, Product3/1, Product1/1, Product/1
  Selector2/1 -> Sum3/2
  Sum3/1 -> Gain2/1
  Gain2/1 -> Sum5/1
  Sum5/1 -> Product2/2
  Product2/1 -> Integrator2/1
  Integrator2/1 -> [v_beta], Product3/2, Sum3/1, Sum6/1
  Product3/1 -> Integrator3/1
  Integrator3/1 -> [qv_beta], Sum5/2
  Sum2/1 -> Mux/1
  Sum6/1 -> Mux/2
  Constant/1 -> Mux/3
  Mux/1 -> Zero-Order Hold2/1
  Zero-Order Hold2/1 -> Ualphbet0/1
  abc to Alpha-Beta-Zero/1 -> Gain/1
  [qv_beta] -> Sum2/2
  [qv_alpha] -> Sum6/2

== system Kundur_BESS_STA_Nov14_2021a_v2_2021a/Area 2/BESS/Support Control/VI with STA/STA-PLL/Quadrature ==
  Uabc : Inport
  w : Inport  Port=2
  Constant : Constant  Value=0
  Divide : Product  Inputs=*/
  Gain : Gain  Gain=1/1000
  Mux : Mux  Inputs=3
  Saturation : Saturate  UpperLimit=62*2*pi  LowerLimit=59*2*pi
  Scope1 : Scope  NumInputPorts=2
  Selector : Selector  InputPortWidth=3  IndexOptions=Index vector (dialog)  Indices=1  OutputSizes=1
  State-Space : StateSpace  A=[-42e3,1,0;-586e6,0,1;-2712e9,0,0]  B=[42e3;586e6;2712e9]  C=[0,1,0]  D=[0]  InitialCondition=0
  Transfer Fcn1 : TransferFcn  Denominator=[1/(1200*2*pi)^2,2*0.1/(1200*2*pi),1]
  Zero-Order Hold2 : ZeroOrderHold  SampleTime=sampling_k
  abc to Alpha-Beta-Zero : spsabctoAlphaBetaZeroLib/abc to Alpha-Beta-Zero
  Ualphbet0 : Outport
  wires:
  Uabc/1 -> Gain/1
  Gain/1 -> abc to Alpha-Beta-Zero/1
  Zero-Order Hold2/1 -> Ualphbet0/1
  abc to Alpha-Beta-Zero/1 -> Selector/1
  Constant/1 -> Mux/3
  Mux/1 -> Zero-Order Hold2/1
  Transfer Fcn1/1 -> Scope1/2, Mux/2, State-Space/1
  State-Space/1 -> Divide/1
  w/1 -> Saturation/1
  Saturation/1 -> Divide/2
  Divide/1 -> Scope1/1, Mux/1
  Selector/1 -> Transfer Fcn1/1

== system Kundur_BESS_STA_Nov14_2021a_v2_2021a/Area 2/BESS/Support Control/VI with STA/STA-PLL/Wrap ==
  phi : Inport
  Constant : Constant  Value=pi
  Constant1 : Constant  Value=2*pi
  Divide : Product  Inputs=*/
  Floor : Rounding
  Product : Product
  Sum : Sum  Inputs=|+-
  Sum1 : Sum  Inputs=|+-
  Sum2 : Sum  Inputs=|+-
  w_phi : Outport
  wires:
  phi/1 -> Sum/1
  Constant/1 -> Sum2/2, Sum/2
  Sum/1 -> Divide/1, Sum1/1
  Constant1/1 -> Product/2, Divide/2
  Divide/1 -> Floor/1
  Floor/1 -> Product/1
  Product/1 -> Sum1/2
  Sum1/1 -> Sum2/1
  Sum2/1 -> w_phi/1

== system Kundur_BESS_STA_Nov14_2021a_v2_2021a/Area 2/BESS/Support Control/VI with STA/STA-PLL/filt1 ==
  u : Inport
  Discrete Transfer Fcn1 : DiscreteTransferFcn  Numerator=flt_rocof_num  Denominator=flt_rocof_den
  uf : Outport
  wires:
  Discrete Transfer Fcn1/1 -> uf/1
  u/1 -> Discrete Transfer Fcn1/1

== system Kundur_BESS_STA_Nov14_2021a_v2_2021a/Area 2/BESS/Support Control/VI with STA/STA-PLL/filt3 ==
  u : Inport
  Discrete Transfer Fcn1 : DiscreteTransferFcn  Numerator=flt_rocof_num  Denominator=flt_rocof_den
  uf : Outport
  wires:
  u/1 -> Discrete Transfer Fcn1/1
  Discrete Transfer Fcn1/1 -> uf/1

== system Kundur_BESS_STA_Nov14_2021a_v2_2021a/Area 2/BESS/Support Control/VI with STA/STA-PLL/filt4 ==
  u : Inport
  Discrete Transfer Fcn1 : DiscreteTransferFcn  Numerator=flt_rocof_a_num  Denominator=flt_rocof_a_den
  Discrete Transfer Fcn2 : DiscreteTransferFcn  Numerator=flt_rocof_b_num  Denominator=flt_rocof_b_den
  Discrete Transfer Fcn3 : DiscreteTransferFcn  Numerator=flt_rocof_a_num  Denominator=flt_rocof_a_den
  Discrete Transfer Fcn4 : DiscreteTransferFcn  Numerator=flt_rocof_b_num  Denominator=flt_rocof_b_den
  uf : Outport
  wires:
  Discrete Transfer Fcn4/1 -> uf/1
  Discrete Transfer Fcn3/1 -> Discrete Transfer Fcn4/1
  Discrete Transfer Fcn2/1 -> Discrete Transfer Fcn3/1
  Discrete Transfer Fcn1/1 -> Discrete Transfer Fcn2/1
  u/1 -> Discrete Transfer Fcn1/1

== matlab function Kundur_BESS_STA_Nov14_2021a_v2_2021a/Area 2/Aggregator1 ==
  data: Plqg input; P output; Qlqg input; Temp input; Smax input; SOC input; Temp_max input; Q output; beta input; fk input; Vk input; fref input; Vref input; DBf input; DBv input; deltaf output; deltaV output; contingency output; time input; timeevent input
function [P, Q, deltaf, deltaV, contingency] = fcn(Plqg, Qlqg, Temp, Smax, SOC, Temp_max, beta, fk, Vk, fref , Vref, DBf, DBv, time, timeevent)

sizePbess=size(Smax);
P= zeros(sizePbess(1),1);
Q= zeros(sizePbess(1),1);
Qmax= zeros(sizePbess(1),1);
Smaxtotal=0;
Qtotal=0;
SOCtotal=0;
Slqg=sqrt(Plqg*Plqg+Qlqg*Qlqg);
deltaf= abs(fk-fref);
deltaV= abs(Vk-Vref);

for i=1:sizePbess(1)%%For each bess the next senstenses are executed, Pbess is the maximum power available in the ith bess.
    if (SOC(i)<0.7 && SOC(i)>0.3 && Temp(i)<Temp_max)
        Smaxtotal=Smaxtotal+Smax(i);
        SOCtotal=SOCtotal+SOC(i);
    end
end

if Smaxtotal>Slqg
    Parea=Plqg;% If the total bess in this area can inject the requested power, so execute the next lines 
    Qarea=Qlqg;
else %if the total bess capacity is smaller than the power requested, so ask if this power is at less greater than P requested
        Parea=(Smaxtotal/Slqg)*Plqg;
        
        %Parea=Smaxtotal;%The total BESS's capacity is smaller than the P requested
        %Qarea=0;
        Qarea=sqrt(Smaxtotal*Smaxtotal-Parea*Parea);
        if Qlqg<0
            Qarea=-Qarea;
        end
end

%%
for i=1:sizePbess(1)%%For each bess the next senstenses are executed, Pbess is the maximum power available in the ith bess.
    P(i)= (beta*(Smax(i)/Smaxtotal)+(1-beta)*(SOC(i)/SOCtotal))*Parea; %gives priority to inject active power. 
    Qmax(i)=sqrt(Smax(i)*Smax(i)-P(i)*P(i));
    Qtotal=Qtotal+Qmax(i);

 
    if ( SOC(i)<0.7 && SOC(i)>0.3 && Temp(i)<Temp_max  &&  (deltaV>DBv || deltaf>DBf) && time>(timeevent+0.1) && deltaV<0.5) 
        contingency=1;  
    elseif (deltaV<DBv && deltaf<DBf)
        contingency=0;
    else 
        contingency=0;
    end
end

for i=1:sizePbess(1)%%For each bess the next senstenses are executed, Pbess is the maximum power available in the ith bess.
    Q(i)=(Qmax(i)/Qtotal)*Qarea;
end

== matlab function Kundur_BESS_STA_Nov14_2021a_v2_2021a/Area 1/BESS2 /MATLAB Function ==
  data: u input; y1 output; y2 output; y3 output
function [y1, y2, y3] = sine_funtion(u)

y1 = sin(2*pi*60*u);
y2 = sin(2*pi*60*u+2*pi/3);
y3 = sin(2*pi*60*u+4*pi/3);

== matlab function Kundur_BESS_STA_Nov14_2021a_v2_2021a/Area 1/BESS2 /MATLAB Function1 ==
  data: P input; id output; Q input; vd input; iq output
function [id, iq]= fcn(P, Q, vd)

id = (2*P)/(3*vd);
iq = -(2*Q)/(3*vd);

== matlab function Kundur_BESS_STA_Nov14_2021a_v2_2021a/Area 1/Aggregator ==
  data: Plqg input; P output; Qlqg input; Temp input; Smax input; SOC input; Temp_max input; Q output; beta input; fk input; Vk input; fref input; Vref input; DBf input; DBv input; deltaf output; deltaV output; contingency output; time input; timeevent input
function [P, Q, deltaf, deltaV, contingency] = fcn(Plqg, Qlqg, Temp, Smax, SOC, Temp_max, beta, fk, Vk, fref , Vref, DBf, DBv, time, timeevent)

sizePbess=size(Smax);
P= zeros(sizePbess(1),1);
Q= zeros(sizePbess(1),1);
Qmax= zeros(sizePbess(1),1);
Smaxtotal=0;
Qtotal=0;
SOCtotal=0;
Slqg=sqrt(Plqg*Plqg+Qlqg*Qlqg);
deltaf= abs(fk-fref);
deltaV= abs(Vk-Vref);

for i=1:sizePbess(1)%%For each bess the next senstenses are executed, Pbess is the maximum power available in the ith bess.
    if (SOC(i)<0.7 && SOC(i)>0.3 && Temp(i)<Temp_max)
        Smaxtotal=Smaxtotal+Smax(i);
        SOCtotal=SOCtotal+SOC(i);
    end
end

if Smaxtotal>Slqg
    Parea=Plqg;% If the total bess in this area can inject the requested power, so execute the next lines 
    Qarea=Qlqg;
else %if the total bess capacity is smaller than the power requested, so ask if this power is at less greater than P requested
        Parea=(Smaxtotal/Slqg)*Plqg;
        
        %Parea=Smaxtotal;%The total BESS's capacity is smaller than the P requested
        %Qarea=0;
        Qarea=sqrt(Smaxtotal*Smaxtotal-Parea*Parea);
        if Qlqg<0
            Qarea=-Qarea;
        end
end

%%
for i=1:sizePbess(1)%%For each bess the next senstenses are executed, Pbess is the maximum power available in the ith bess.
    P(i)= (beta*(Smax(i)/Smaxtotal)+(1-beta)*(SOC(i)/SOCtotal))*Parea; %gives priority to inject active power. 
    Qmax(i)=sqrt(Smax(i)*Smax(i)-P(i)*P(i));
    Qtotal=Qtotal+Qmax(i);

 
    if ( SOC(i)<0.7 && SOC(i)>0.3 && Temp(i)<Temp_max  &&  (deltaV>DBv || deltaf>DBf) && time>(timeevent+0.1) && deltaV<0.5) 
        contingency=1;  
    elseif (deltaV<=DBv && deltaf<=DBf)
        contingency=0;
    else 
        contingency=0;
    end
end

for i=1:sizePbess(1)%%For each bess the next senstenses are executed, Pbess is the maximum power available in the ith bess.
    Q(i)=(Qmax(i)/Qtotal)*Qarea;
end

== matlab function Kundur_BESS_STA_Nov14_2021a_v2_2021a/MATLAB Function ==
  data: event input; y output; time input
function y = fcn(event, time)

if event>time
    y=1;
else
    y=0;
end

== matlab function Kundur_BESS_STA_Nov14_2021a_v2_2021a/Area 1/BESS/MATLAB Function ==
  data: u input; y1 output; y2 output; y3 output
function [y1, y2, y3] = sine_funtion(u)

y1 = sin(2*pi*60*u);
y2 = sin(2*pi*60*u+2*pi/3);
y3 = sin(2*pi*60*u+4*pi/3);

== matlab function Kundur_BESS_STA_Nov14_2021a_v2_2021a/Area 1/BESS/MATLAB Function1 ==
  data: P input; id output; Q input; vd input; iq output
function [id, iq]= fcn(P, Q, vd)

id = (2*P)/(3*vd);
iq = -(2*Q)/(3*vd);
